simulink model "fuzzy"  (R2024a)
settings: Solver=FixedStepAuto  StartTime=0.0  StopTime=250  FixedStep=1e-2  RelTol=1e-3
InitFcn:
  | % close;
  | % % % z
  | k_p_z = -4;
  | k_i_z = -.5;
  | k_d_z = -8;
  | k_a_z = -2;
  | % %
  | % % % psi
  | k_p_psi = 5.84;
  | k_i_psi = 0;
  | k_d_psi = .836;
  | k_a_psi = 0;
  | % %
  | % % phi
  | k_p_phi = 1;
  | k_d_phi = 0.32;
  | %
  | % % tt
  | k_p_tt = 1;
  | k_d_tt = .302;
  | %
  | % % x
  | k_p_x = -5.99;
  | k_i_x = -2.8;
  | k_d_x = -1.244;
  | k_a_x = -7.94;
  | %
  | % % y
  | k_p_y = 5.99;
  | k_i_y = 2.8;
  | k_d_y = 1.244;
  | k_a_y = 7.94;
StopFcn:
  | plot3(x,y,-z,['b','-'],x_g,y_g,-z_g,['r','--'],'LineWidth',1.25);
  | xlabel('x');
  | ylabel('y');
  | zlabel('z');
  | grid on;
undefined symbols (not defined in the file): k_a_phi, k_a_tt, k_i_phi, k_i_tt
libraries: fuzblock x6, simulink x6
settings Model: Creator=luand  LastModifiedBy=luand
settings DataIOCC: ReturnWorkspaceOutputs=off

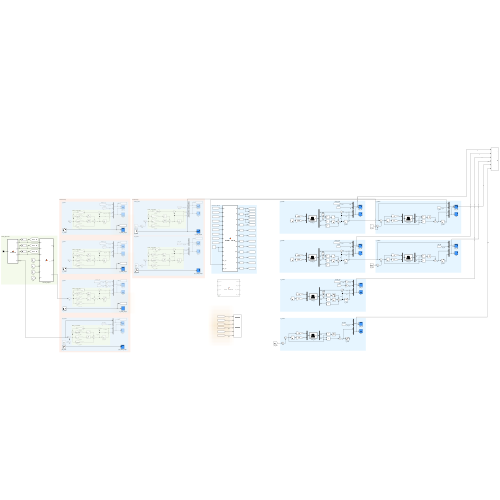
[thumbnail: Simulink's stored preview of the top-level diagram]
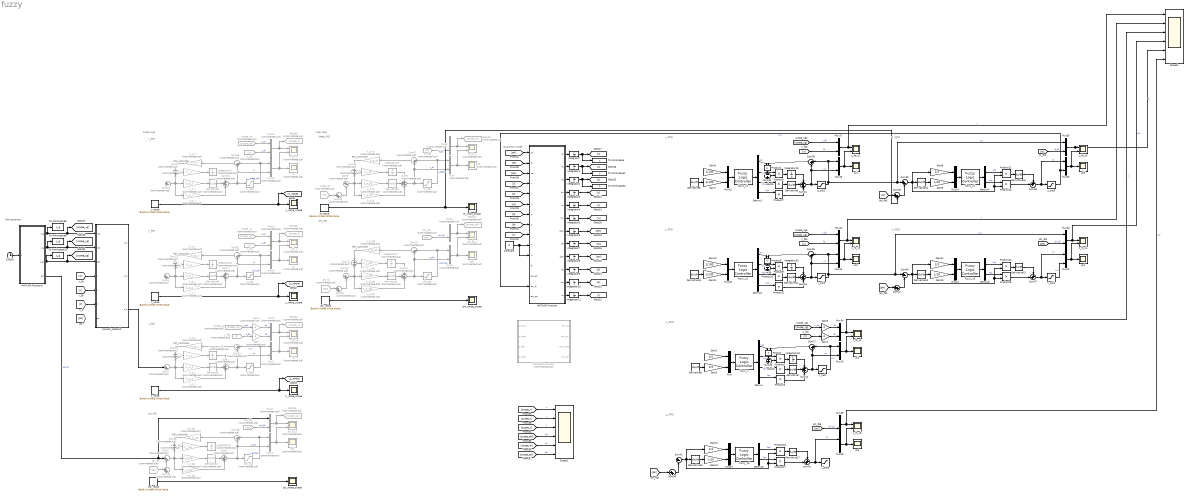
== system fuzzy ==
  note: Path generate
  note: Inner loop
  note: z_PID
  note: PID_controller
  note: PID_controller
  note: psi_PID
  note: Quadrotor Model
  note: PID_controller
  note: PID_controller
  note: PID_controller
  note: PID_controller
  note: theta_PID
  note: phi_PID
  note: Outer loop
  note: y_PID
  note: x_PID
  note: z_FPID
  note: x_FPID
  note: y_FPID
  note: z_FPID
  note: z_FPID
  note: z_FPID
  Clock5 : Clock
  Constant : Constant  Value=0
  Demux : Demux
  Demux1 : Demux
  Demux2 : Demux
  Demux3 : Demux  Outputs=2
  Demux4 : Demux  Outputs=2
  Demux5 : Demux  Outputs=2
  Derivative{,1..5} (6 alike) : Derivative  Commented=on
  Derivative{6..17} (12 alike) : Derivative
  Gain : Gain  Commented=on  Gain=-1
  Gain1 : Gain  Commented=on  Gain=-1
  Gain{6..7,10..11} (4 alike) : Gain  Gain=1/100
  Gain12 : Gain  Gain=1/3
  Gain13 : Gain  Gain=1/10
  Gain14 : Gain  Gain=1/3
  Gain15 : Gain  Gain=1/10
  Gain2 : Gain  Gain=1/5
  Gain3 : Gain  Gain=1/5
  Gain4 : Gain  Gain=-1
  Gain5 : Gain  Gain=-1
  Gain8 : Gain  Gain=1/3
  Gain9 : Gain  Gain=1/10
  Goto24 : Goto  Commented=on  GotoTag=scope_phi
  Goto25 : Goto  Commented=on  GotoTag=scope_y
  Goto26 : Goto  Commented=on  GotoTag=scope_tt
  Goto28 : Goto  Commented=on  GotoTag=scope_psi
  Goto30 : Goto  Commented=on  GotoTag=scope_x
  Goto34 : Goto  Commented=on  GotoTag=scope_z
  Integrator{,1,3..5} (5 alike) : Integrator  LimitOutput=on  UpperSaturationLimit=10000  LowerSaturationLimit=-10000
  Integrator{8..11} (4 alike) : Integrator  LimitOutput=on  UpperSaturationLimit=100  LowerSaturationLimit=-100
  Integrator{12..15,17} (5 alike) : Integrator  Commented=on  LimitOutput=on  UpperSaturationLimit=1000  LowerSaturationLimit=-1000
  Integrator16 : Integrator  Commented=on
  Integrator{6..7,18..20} (5 alike) : Integrator  LimitOutput=on  UpperSaturationLimit=1000  LowerSaturationLimit=-1000
  Integrator2 : Integrator  LimitOutput=on  UpperSaturationLimit=0  LowerSaturationLimit=-1000
  MATLAB Function : MATLAB Function  TreatAsAtomicUnit=on
  MATLAB Function1 : MATLAB Function  Commented=on  TreatAsAtomicUnit=on
  MATLAB Function2 : MATLAB Function  TreatAsAtomicUnit=on
  Mux{,13..29} (18 alike) : Mux  Inputs=2
  Mux{1..12} (12 alike) : Mux  Commented=on  Inputs=2
  Product{,1..17} (18 alike) : Product
  Scope1 : Scope  NumInputPorts=6
  Scope2 : Scope  NumInputPorts=6
  Sum{1,3,7,9,11,33} (6 alike) : Sum  Commented=on  Inputs=+++
  Sum{2,4,6,8,10,12} (6 alike) : Sum  Commented=on  Inputs=|+-
  Sum13 : Sum  Commented=on  Inputs=++|
  Sum14 : Sum  Inputs=+++
  Sum{15,19,22,27,29,32} (6 alike) : Sum  Commented=on  Inputs=|-+
  Sum16 : Sum  Commented=on  Inputs=-|+
  Sum17 : Sum  Inputs=|-+
  Sum18 : Sum  Commented=on  Inputs=+|+
  Sum20 : Sum  Inputs=-|+
  Sum21 : Sum  Commented=on  Inputs=+|+
  Sum23 : Sum  Commented=on  Inputs=|++
  Sum24 : Sum  Inputs=+++
  Sum25 : Sum  Commented=on  Inputs=|++
  Sum26 : Sum  Commented=on  Inputs=+|+
  Sum28 : Sum  Inputs=|-+
  Sum30 : Sum  Inputs=-|+
  Sum31 : Sum  Commented=on  Inputs=-|+
  Sum34 : Sum  Inputs=+++
  Sum35 : Sum  Inputs=|-+
  Sum36 : Sum  Inputs=-|+
  Sum37 : Sum  Inputs=++|
  Sum38 : Sum  Inputs=++|
  Sum39 : Sum  Inputs=|+-
  Sum40 : Sum  Inputs=|+-
  Sum41 : Sum  Inputs=++|
  Sum42 : Sum  Inputs=|+-
  Sum45 : Sum  Inputs=|++
  Sum46 : Sum  Inputs=|++
  Sum47 : Sum  Inputs=|++
  Sum5 : Sum  Commented=on  Inputs=-|+
  To Workspace : ToWorkspace  VariableName=x  SampleTime=-1
      settings: Save2DSignal=2-D array (concatenate along first dimension)
  To Workspace1 : ToWorkspace  VariableName=y  SampleTime=-1
      settings: Save2DSignal=2-D array (concatenate along first dimension)
  To Workspace10 : ToWorkspace  VariableName=z_g  SampleTime=-1
      settings: Save2DSignal=2-D array (concatenate along first dimension)
  To Workspace2 : ToWorkspace  VariableName=z  SampleTime=-1
      settings: Save2DSignal=2-D array (concatenate along first dimension)
  To Workspace8 : ToWorkspace  VariableName=x_g  SampleTime=-1
      settings: Save2DSignal=2-D array (concatenate along first dimension)
  To Workspace9 : ToWorkspace  VariableName=y_g  SampleTime=-1
      settings: Save2DSignal=2-D array (concatenate along first dimension)
  convert_setpoint : MATLAB Function  TreatAsAtomicUnit=on
  fuzzy_z : fuzblock/Fuzzy Logic  Controller  FIS='fuzzy_z.fis'  OutputSampleNumber=11  DataType=double  FuzzifiedInputs=off  RuleFiringStrengths=off  RuleOutputs=off  AggregatedOutputs=off  SimulateUsing=Interpreted execution  OutOfRangeInputValueMessage=warning  NoRuleFiredMessage=warning  EmptyOutputFuzzySetMessage=warning
  fuzzy_z1 : fuzblock/Fuzzy Logic  Controller  FIS='fuzzy_x.fis'  OutputSampleNumber=11  DataType=double  FuzzifiedInputs=off  RuleFiringStrengths=off  RuleOutputs=off  AggregatedOutputs=off  SimulateUsing=Interpreted execution  OutOfRangeInputValueMessage=warning  NoRuleFiredMessage=warning  EmptyOutputFuzzySetMessage=warning
  fuzzy_z2 : fuzblock/Fuzzy Logic  Controller  FIS='fuzzy_y.fis'  OutputSampleNumber=11  DataType=double  FuzzifiedInputs=off  RuleFiringStrengths=off  RuleOutputs=off  AggregatedOutputs=off  SimulateUsing=Interpreted execution  OutOfRangeInputValueMessage=warning  NoRuleFiredMessage=warning  EmptyOutputFuzzySetMessage=warning
  fuzzy_z3 : fuzblock/Fuzzy Logic  Controller  FIS='fuzzy_phi.fis'  OutputSampleNumber=101  DataType=double  FuzzifiedInputs=off  RuleFiringStrengths=off  RuleOutputs=off  AggregatedOutputs=off  SimulateUsing=Interpreted execution  OutOfRangeInputValueMessage=warning  NoRuleFiredMessage=warning  EmptyOutputFuzzySetMessage=warning
  fuzzy_z4 : fuzblock/Fuzzy Logic  Controller  FIS='fuzzy_tt.fis'  OutputSampleNumber=101  DataType=double  FuzzifiedInputs=off  RuleFiringStrengths=off  RuleOutputs=off  AggregatedOutputs=off  SimulateUsing=Interpreted execution  OutOfRangeInputValueMessage=warning  NoRuleFiredMessage=warning  EmptyOutputFuzzySetMessage=warning
  fuzzy_z5 : fuzblock/Fuzzy Logic  Controller  FIS='fuzzy_psi.fis'  OutputSampleNumber=101  DataType=double  FuzzifiedInputs=off  RuleFiringStrengths=off  RuleOutputs=off  AggregatedOutputs=off  SimulateUsing=Interpreted execution  OutOfRangeInputValueMessage=warning  NoRuleFiredMessage=warning  EmptyOutputFuzzySetMessage=warning
  k_a_phi : Gain  Commented=on  Gain=k_a_phi
  k_a_psi : Gain  Commented=on  Gain=k_a_psi
  k_a_tt : Gain  Commented=on  Gain=k_a_tt
  k_a_x : Gain  Commented=on  Gain=k_a_x
  k_a_y : Gain  Commented=on  Gain=k_a_y
  k_a_z : Gain  Commented=on  Gain=k_a_z
  k_d_phi : Gain  Commented=on  Gain=k_d_phi
  k_d_psi : Gain  Commented=on  Gain=k_d_psi
  k_d_tt : Gain  Commented=on  Gain=k_d_tt
  k_d_x : Gain  Commented=on  Gain=k_d_x
  k_d_y : Gain  Commented=on  Gain=k_d_y
  k_d_z : Gain  Commented=on  Gain=k_d_z
  k_i_phi : Gain  Commented=on  Gain=k_i_phi
  k_i_psi : Gain  Commented=on  Gain=k_i_psi
  k_i_tt : Gain  Commented=on  Gain=k_i_tt
  k_i_x : Gain  Commented=on  Gain=k_i_x
  k_i_y : Gain  Commented=on  Gain=k_i_y
  k_i_z : Gain  Commented=on  Gain=k_i_z
  k_p_phi : Gain  Commented=on  Gain=k_p_phi
  k_p_psi : Gain  Commented=on  Gain=k_p_psi
  k_p_tt : Gain  Commented=on  Gain=k_p_tt
  k_p_x : Gain  Commented=on  Gain=k_p_x
  k_p_y : Gain  Commented=on  Gain=k_p_y
  k_p_z : Gain  Commented=on  Gain=k_p_z
  phi_fb : From  Commented=on  GotoTag=phi
  phi_fb1 : From  Commented=on  GotoTag=phi
  phi_fb_u : Scope  Commented=on  NumInputPorts=2
  phi_noise : simulink/Sources/Band-Limited White Noise  Cov=[0.001]  Ts=0.1  seed=[23341]
  phi_noise_scope : Scope
  phi_sat : Saturate  Commented=on  UpperLimit=100  LowerLimit=-100
  psi_fb : From  Commented=on  GotoTag=psi
  psi_fb1 : From  Commented=on  GotoTag=psi
  psi_fb_u : Scope  Commented=on  NumInputPorts=2
  psi_noise : simulink/Sources/Band-Limited White Noise  Cov=[0.0005]  Ts=0.1  seed=[12424]
  psi_noise_scope : Scope
  psi_sat : Saturate  Commented=on  UpperLimit=50  LowerLimit=-50
  scope_xg : From  Commented=on  GotoTag=scope_xg
  scope_yg : From  Commented=on  GotoTag=scope_yg
  scope_zg : From  Commented=on  GotoTag=scope_zg
  theta_fb : From  Commented=on  GotoTag=tt
  tt_fb1 : From  Commented=on  GotoTag=tt
  tt_fb_u : Scope  Commented=on  NumInputPorts=2
  tt_noise : simulink/Sources/Band-Limited White Noise  Cov=[0.001]  Ts=0.1  seed=[23341]
  tt_noise_scope : Scope
  tt_sat : Saturate  Commented=on  UpperLimit=100  LowerLimit=-100
  uphi : Scope  Commented=on
  upsi : Scope  Commented=on
  utt : Scope  Commented=on
  ux : Scope  Commented=on
  uy : Scope  Commented=on
  uz : Scope  Commented=on
  uz{1..6} (6 alike) : Scope
  x_fb1 : From  Commented=on  GotoTag=x
  x_fb_u : Scope  Commented=on  NumInputPorts=2
  x_noise : simulink/Sources/Band-Limited White Noise  Cov=[0.0001]  Ts=0.1  seed=[23341]
  x_noise_scope : Scope
  x_sat : Saturate  Commented=on  UpperLimit=pi/2  LowerLimit=-pi/2
  y_fb1 : From  Commented=on  GotoTag=y
  y_fb_u : Scope  Commented=on  NumInputPorts=2
  y_noise : simulink/Sources/Band-Limited White Noise  Cov=[0.0001]  Ts=0.1  seed=[24432]
  y_noise_scope : Scope
  y_sat : Saturate  Commented=on  UpperLimit=pi/2  LowerLimit=-pi/2
  z_fb1 : From  Commented=on  GotoTag=z
  z_fb_u : Scope  Commented=on  NumInputPorts=2
  z_fb_u{1..6} (6 alike) : Scope  NumInputPorts=2
  z_noise : simulink/Sources/Band-Limited White Noise  Cov=[0.01]  Ts=0.1  seed=[55123]
  z_noise_scope : Scope
  z_sat : Saturate  Commented=on  UpperLimit=40  LowerLimit=0
  z_sat1 : Saturate  UpperLimit=40  LowerLimit=0
  z_sat2 : Saturate  UpperLimit=pi/15  LowerLimit=-pi/15
  z_sat3 : Saturate  UpperLimit=pi/15  LowerLimit=-pi/15
  z_sat4 : Saturate  UpperLimit=100  LowerLimit=-100
  z_sat5 : Saturate  UpperLimit=100  LowerLimit=-100
  z_sat6 : Saturate  UpperLimit=100  LowerLimit=-100
  wires:
  k_a_phi/1 -> Sum21/1
  phi_fb/1 -> Sum23/1
  Sum23/1 -> Sum10/2
  Sum11/1 -> Mux5/2, Sum22/2, phi_sat/1  "u_phi"
  k_d_phi/1 -> Derivative2/1
  phi_fb1/1 -> Mux6/2  "phi_fb"
  Mux5/1 -> uphi/1, phi_fb_u/2
  Mux6/1 -> phi_fb_u/1, Goto24/1
  x_sat/1 -> Mux12/1, Sum29/1  "theta_ref"
  Sum21/1 -> k_i_phi/1
  [r] -> MATLAB Function/9(r)
  MATLAB Function2/4(psi) -> Mux3/1, Sum2/1  "psi_sp"
  phi_noise/1 -> phi_noise_scope/1
  Integrator8/1 -> [psi]
  Sum13/1 -> Sum2/2
  Sum19/1 -> k_a_psi/1
  psi_fb1/1 -> Mux3/2  "psi_fb"
  MATLAB Function/11(dq) -> Integrator10/1
  Mux4/1 -> upsi/1, psi_fb_u/2
  Constant/1 -> MATLAB Function/11(fy), MATLAB Function/10(fx)
  k_a_psi/1 -> Sum18/1
  Mux1/1 -> uz/1, z_fb_u/2
  Mux3/1 -> psi_fb_u/1, Goto28/1
  k_p_psi/1 -> Sum3/3
  Derivative1/1 -> Sum3/2
  Gain/1 -> Mux2/2  "fb"
  Integrator5/1 -> [w]
  [tt] -> MATLAB Function/2(tt)
  Sum22/1 -> k_a_phi/1
  k_p_phi/1 -> Sum11/3
  Integrator/1 -> To Workspace/1, [x]
  psi_sat/1 -> Sum19/1, Mux4/1  "u_psisat"
  MATLAB Function/4(du) -> Integrator3/1
  k_d_psi/1 -> Derivative1/1
  Sum16/1 -> k_i_z/1
  Integrator12/1 -> Sum1/1
  k_a_z/1 -> Sum16/1
  Mux2/1 -> Goto34/1, z_fb_u/1
  Gain1/1 -> Mux2/1  "sp"
  [phi] -> MATLAB Function/1(phi)
  k_d_z/1 -> Derivative/1
  z_noise/1 -> [z_noise], z_noise_scope/1
  Integrator10/1 -> [q]
  k_i_z/1 -> Integrator12/1
  Sum1/1 -> Mux1/2, Sum15/2, z_sat/1  "uz"
  psi_fb/1 -> Sum13/1
  Sum18/1 -> k_i_psi/1
  Derivative2/1 -> Sum11/2
  [psi] -> MATLAB Function/3(psi)
  k_i_phi/1 -> Integrator17/1
  phi_sat/1 -> Mux5/1, Sum22/1  "u_phisat"
  k_i_tt/1 -> Integrator16/1
  k_i_y/1 -> Integrator15/1
  z_sat/1 -> Mux1/1, Sum15/1  "u_z"
  [p] -> MATLAB Function/7(p)
  MATLAB Function/1(dx) -> Integrator/1
  Integrator7/1 -> [tt]
  Sum2/1 -> Sum18/2, k_d_psi/1, k_p_psi/1
  Integrator1/1 -> To Workspace1/1, [y]
  MATLAB Function/2(dy) -> Integrator1/1
  k_i_psi/1 -> Integrator13/1
  Integrator3/1 -> [u]
  Sum3/1 -> psi_sat/1, Sum19/2, Mux4/2  "u_psi"
  Integrator2/1 -> To Workspace2/1, [z]
  [w] -> MATLAB Function/6(w)
  Integrator11/1 -> [r]
  Integrator9/1 -> [p]
  [u] -> MATLAB Function/4(u)
  Integrator6/1 -> [phi]
  MATLAB Function/5(dv) -> Integrator4/1
  psi_noise/1 -> psi_noise_scope/1
  MATLAB Function/6(dw) -> Integrator5/1
  z_fb1/1 -> Gain/1  "z_fb"
  Integrator4/1 -> [v]
  MATLAB Function/12(dr) -> Integrator11/1
  MATLAB Function/9(dpsi) -> Integrator8/1
  [q] -> MATLAB Function/8(q)
  Sum10/1 -> k_d_phi/1, Sum21/2, k_p_phi/1
  [v] -> MATLAB Function/5(v)
  MATLAB Function/10(dp) -> Integrator9/1
  MATLAB Function/8(dtt) -> Integrator7/1
  Sum15/1 -> k_a_z/1
  MATLAB Function/3(dz) -> Integrator2/1
  MATLAB Function/7(dphi) -> Integrator6/1
  Integrator17/1 -> Sum11/1
  theta_fb/1 -> Sum25/1
  Sum25/1 -> Sum8/2
  Integrator16/1 -> Sum9/1
  k_p_tt/1 -> Sum9/3
  Sum26/1 -> k_i_tt/1
  k_d_tt/1 -> Derivative3/1
  Derivative3/1 -> Sum9/2
  k_a_tt/1 -> Sum26/1
  Sum27/1 -> k_a_tt/1
  tt_sat/1 -> Mux7/1, Sum27/1  "u_ttsat"
  y_sat/1 -> Mux9/1, Sum32/1  "phi_ref"
  Mux8/1 -> Goto26/1, tt_fb_u/1
  Mux7/1 -> utt/1, tt_fb_u/2
  tt_fb1/1 -> Mux8/2  "tt_fb"
  Sum9/1 -> Mux7/2, Sum27/2, tt_sat/1  "u_tt"
  tt_noise/1 -> Sum46/2, tt_noise_scope/1
  Sum8/1 -> k_d_tt/1, Sum26/2, k_p_tt/1
  Integrator13/1 -> Sum3/1
  Clock5/1 -> MATLAB Function2/1(t)
  k_d_y/1 -> Derivative4/1
  Integrator15/1 -> Sum7/1
  k_p_y/1 -> Sum7/3
  Sum31/1 -> k_i_y/1
  k_a_y/1 -> Sum31/1
  Sum7/1 -> Mux9/2, Sum32/2, y_sat/1  "uy"
  Sum32/1 -> k_a_y/1
  y_noise/1 -> [y_noise], y_noise_scope/1
  x_noise/1 -> [x_noise], x_noise_scope/1
  Sum29/1 -> k_a_x/1
  Sum33/1 -> x_sat/1, Sum29/2, Mux12/2  "ux"
  k_a_x/1 -> Sum5/1
  Sum5/1 -> k_i_x/1
  k_p_x/1 -> Sum33/3
  Integrator14/1 -> Sum33/1
  k_d_x/1 -> Derivative5/1
  k_i_x/1 -> Integrator14/1
  y_fb1/1 -> Mux10/2  "y_fb"
  Mux10/1 -> Goto25/1, y_fb_u/1
  Mux9/1 -> uy/1, y_fb_u/2
  Mux11/1 -> x_fb_u/1, Goto30/1
  Mux12/1 -> ux/1, x_fb_u/2
  x_fb1/1 -> Mux11/2  "x_fb"
  [scope_x] -> Scope1/1  "x"
  [scope_y] -> Scope1/2  "y"
  [scope_z] -> Scope1/3  "z"
  [scope_psi] -> Scope1/6  "psi"
  [scope_phi] -> Scope1/4  "phi"
  [scope_tt] -> Scope1/5  "tt"
  Derivative4/1 -> Sum7/2
  Derivative5/1 -> Sum33/2
  MATLAB Function2/1(x_g) -> [scope_xg], convert_setpoint/1(xsp), To Workspace8/1
  MATLAB Function2/2(y_g) -> [scope_yg], convert_setpoint/2(ysp), To Workspace9/1
  MATLAB Function2/3(z_g) -> [scope_zg], convert_setpoint/3(zsp), To Workspace10/1
  scope_xg/1 -> Mux11/1  "x_sp"
  scope_zg/1 -> Gain1/1  "z_sp"
  scope_yg/1 -> Mux10/1  "y_sp"
  [x] -> convert_setpoint/4(x)
  [y] -> convert_setpoint/5(y)
  [z] -> convert_setpoint/6(z)
  Sum4/1 -> Sum16/2, k_p_z/1, k_d_z/1
  Sum12/1 -> Sum5/2, k_p_x/1, k_d_x/1
  Sum6/1 -> Sum31/2, k_p_y/1, k_d_y/1
  Derivative/1 -> Sum1/2
  Derivative6/1 -> Gain3/1
  Gain2/1 -> Mux/1
  Gain3/1 -> Mux/2
  Derivative7/1 -> Sum14/2
  z_sat1/1 -> Mux13/1, Sum17/1  "u_z"
  Sum14/1 -> z_sat1/1, Mux13/2, Sum17/2  "uz"
  Product1/1 -> Integrator18/1
  Product2/1 -> Derivative7/1
  Integrator18/1 -> Sum14/1
  fuzzy_z/1 -> Demux/1
  Product/1 -> Sum20/1
  Demux/3 -> Product2/1  "kdz"
  Demux/4 -> Product3/1  "kpz"
  Product3/1 -> Sum14/3
  Mux/1 -> fuzzy_z/1
  k_p_z/1 -> Sum1/3
  Demux/2 -> Product1/1  "kiz"
  Sum20/1 -> Product1/2
  Demux/1 -> Product/1  "kaz"
  Sum17/1 -> Product/2
  convert_setpoint/3(z_b) -> Sum4/1
  [scope_zg] -> Gain5/1  "x_fb"
  [z] -> Gain4/1
  Gain5/1 -> Mux14/1  "sp"
  Mux14/1 -> Scope2/3, z_fb_u1/1  "z"
  Gain4/1 -> Mux14/2  "fb"
  Mux13/1 -> uz1/1, z_fb_u1/2
  Mux16/1 -> z_fb_u2/2, uz2/1
  [x] -> Mux17/2  "fb"
  Mux17/1 -> Scope2/1, z_fb_u2/1  "x"
  [scope_xg] -> Mux17/1  "x_fb"
  Sum28/1 -> Product4/2
  Demux1/1 -> Product4/1  "kaz"
  Sum30/1 -> Product5/2
  Demux1/2 -> Product5/1  "kiz"
  Mux15/1 -> fuzzy_z1/1
  Product7/1 -> Sum24/3
  Demux1/4 -> Product7/1  "kpz"
  Demux1/3 -> Product6/1  "kdz"
  Product4/1 -> Sum30/1
  fuzzy_z1/1 -> Demux1/1
  Integrator19/1 -> Sum24/1
  Product6/1 -> Derivative9/1
  Product5/1 -> Integrator19/1
  Sum24/1 -> Sum28/2, Mux16/2, z_sat2/1  "uz"
  z_sat2/1 -> Mux26/1, Sum39/1, Mux16/1, Sum28/1  "u_z"
  Derivative9/1 -> Sum24/2
  Gain7/1 -> Mux15/2
  Gain6/1 -> Mux15/1
  Derivative8/1 -> Gain7/1
  Derivative10/1 -> Gain11/1
  Gain10/1 -> Mux18/1
  Gain11/1 -> Mux18/2
  Derivative11/1 -> Sum34/2
  z_sat3/1 -> Mux23/1, Sum40/1, Sum35/1, Mux19/1  "u_z"
  Sum34/1 -> z_sat3/1, Mux19/2, Sum35/2  "uz"
  Product9/1 -> Integrator20/1
  Product10/1 -> Derivative11/1
  Integrator20/1 -> Sum34/1
  fuzzy_z2/1 -> Demux2/1
  Product8/1 -> Sum36/1
  Demux2/3 -> Product10/1  "kdz"
  Demux2/4 -> Product11/1  "kpz"
  Product11/1 -> Sum34/3
  Mux18/1 -> fuzzy_z2/1
  Demux2/2 -> Product9/1  "kiz"
  Sum36/1 -> Product9/2
  Demux2/1 -> Product8/1  "kaz"
  Sum35/1 -> Product8/2
  [scope_yg] -> Mux20/1  "x_fb"
  Mux20/1 -> Scope2/2, z_fb_u3/1  "y"
  [y] -> Mux20/2  "fb"
  Mux19/1 -> uz3/1, z_fb_u3/2
  Mux22/1 -> z_fb_u4/2, uz4/1
  Sum40/1 -> Gain14/1, Derivative12/1, Product14/2, Product15/2
  Mux21/1 -> fuzzy_z3/1
  Demux3/2 -> Product15/1  "kpz"
  Demux3/1 -> Product14/1  "kdz"
  fuzzy_z3/1 -> Demux3/1
  Product14/1 -> Derivative13/1
  Sum37/1 -> Mux22/1, z_sat4/1  "uz"
  z_sat4/1 -> Mux22/2  "u_z"
  Gain15/1 -> Mux21/2
  Gain14/1 -> Mux21/1
  Derivative12/1 -> Gain15/1
  Mux26/1 -> Scope2/5, z_fb_u5/1  "tt"
  Mux23/1 -> Scope2/4, z_fb_u4/1  "phi"
  Derivative13/1 -> Sum37/1
  Product15/1 -> Sum37/2
  Product13/1 -> Sum38/2
  Derivative15/1 -> Sum38/1
  Derivative14/1 -> Gain9/1
  Gain8/1 -> Mux24/1
  Gain9/1 -> Mux24/2
  Sum38/1 -> z_sat5/1, Mux25/1  "uz"
  Product12/1 -> Derivative15/1
  fuzzy_z4/1 -> Demux4/1
  Demux4/1 -> Product12/1  "kdz"
  Demux4/2 -> Product13/1  "kpz"
  Mux24/1 -> fuzzy_z4/1
  Sum39/1 -> Product13/2, Product12/2, Derivative14/1, Gain8/1
  Mux25/1 -> uz5/1, z_fb_u5/2
  z_sat5/1 -> Mux25/2, MATLAB Function/14(tau_tt)  "u_z"
  [tt] -> Mux26/2  "tt_fb"
  [phi] -> Mux23/2  "phi_fb"
  [psi] -> Mux29/2  "phi_fb"
  Product17/1 -> Sum41/2
  Derivative17/1 -> Sum41/1
  Derivative16/1 -> Gain13/1
  Gain12/1 -> Mux27/1
  Gain13/1 -> Mux27/2
  Sum41/1 -> z_sat6/1, Mux28/1  "uz"
  Product16/1 -> Derivative17/1
  fuzzy_z5/1 -> Demux5/1
  Demux5/1 -> Product16/1  "kdz"
  Demux5/2 -> Product17/1  "kpz"
  Mux27/1 -> fuzzy_z5/1
  Sum42/1 -> Product17/2, Product16/2, Derivative16/1, Gain12/1
  Mux28/1 -> uz6/1, z_fb_u6/2
  Mux29/1 -> Scope2/6, z_fb_u6/1  "psi"
  [psi] -> Sum45/1
  Sum45/1 -> Sum42/2
  [tt] -> Sum46/1
  Sum46/1 -> Sum39/2
  [phi] -> Sum47/1
  Sum47/1 -> Sum40/2

== matlab function fuzzy/MATLAB Function1 ==
  data: fthrust output; tau_phi output; tau_theta output; tau_psi output; p_front input; p_back input; p_left input; p_right input
function [fthrust, tau_phi, tau_theta, tau_psi] = Motor_dynamics(p_front, p_back, p_left, p_right)

fthrust = k_thrust*(p_front+p_back+p_left+p_right);
tau_phi = l*k_thrust*(-p_right+p_left);
tau_theta = l*k_thrust*(p_front+p_back);
tau_psi = k_momen*(-p_front-p_back+p_left+p_right);

== matlab function fuzzy/MATLAB Function ==
  data: phi input; tt input; psi input; u input; dx output; v input; w input; p input; q input; r input; fx input; fy input; fz input; tau_phi input; tau_tt input; tau_psi input; dy output; dz output; du output; dv output; dw output; dphi output; dtt output; dpsi output; dp output; dq output; dr output
function [dx,dy,dz,du,dv,dw,dphi,dtt,dpsi,dp,dq,dr]=Dynamics_plustype(phi,tt,psi,u,v,w,p,q,r,fx,fy,fz,tau_phi,tau_tt,tau_psi)

% Eqs. 16-19

M = 1.2;
m = .075;
g = 9.81;
R = .1;
l = .22;

Jx = .4*M*R*R+2*l*l*m;
Jy = .4*M*R*R+2*l*l*m;
Jz = .4*M*R*R+4*l*l*m;

dx = cos(tt)*cos(psi)*u+(sin(phi)*sin(tt)*cos(psi)-cos(phi)*sin(psi))*v+(cos(phi)*sin(tt)*cos(psi)+sin(phi)*sin(psi))*w;
dy = cos(tt)*sin(psi)*u+(sin(phi)*sin(tt)*sin(psi)+cos(phi)*cos(psi))*v+(cos(phi)*sin(tt)*sin(psi)-sin(phi)*cos(psi))*w;
dz = -(sin(tt)*u-sin(phi)*cos(tt)*v-cos(phi)*cos(tt)*w);

du = (r*v-q*w)-g*sin(tt);
dv = (p*w-r*u)+g*cos(tt)*sin(phi);
dw = (q*u-p*v)+g*cos(tt)*cos(phi)-fz/(M+4*m);

dphi = p+sin(phi)*tan(phi)*q+cos(phi)*tan(tt)*r;
dtt  = cos(phi)*q-sin(phi)*r;
dpsi = sin(phi)*q/cos(tt)+cos(phi)*r/cos(tt);

dp = ((Jy-Jz)*q*r+tau_phi)/Jx;
dq = ((Jz-Jx)*p*r+tau_tt)/Jy;
dr = ((Jx-Jy)*q*p+tau_psi)/Jz;

== matlab function fuzzy/MATLAB Function2 ==
  data: t input; x_g output; y_g output; z_g output; psi output
function [x_g,y_g,z_g,psi] = path_ground(t)

% psi = 100-100*exp(-.02*t);
psi = 0;
% psi = sin(.3*t);
% psi = t/2;

% x_g=0;
% y_g=0;
% if t<30
%     z_g = -10;
% elseif t<70
%     z_g = -20;
% elseif t<100
%     z_g = -30;
% else
%     z_g = 0;
% end

% A = 10; % x range
% a = 5; % grid x
% B = 10; % y range
% b = 4; % grid y
% C = 10;% z range 
% coef = .07;
% x_g = (A-.2*exp(-.014*(t-279.4)))*cos(a*coef*t);
% y_g = (B-.2*exp(-.014*(t-279.4)))*sin(b*coef*t);
% z_g = -C*(1-exp(-5*coef*t));%-sin(.3*t)*sin(.3*t);

% z_g = -C*(1-exp(-.03*t));

% A = 20; % x range
% a = 5; % grid x
% B = 20; % y range
% b = 4; % grid y
% C = 10;% z range 
% coef = .07;
% x_g = (10-.2*exp(-.014*(t-279.4)))*cos(a*coef*t);
% y_g = (10-.2*exp(-.014*(t-279.4)))*sin(b*coef*t);
% % z_g = -10; % dont know why step Z work
% % z_g = -(10-.2*exp(-.014*(t-279.4)));
% z_g = -(10-10*exp(-.05*t));

if t<25
    x_g = 1*t/25;
    y_g = 1*t/25;
    z_g = -3-2*t/25;
elseif t<50
    x_g = 1+(t-25)/25;
    y_g = 1;
    z_g = -5-2*(t-25)/25;
elseif t<75
    x_g = 2;
    y_g = 1+(t-50)/25;
    z_g = -7-2*(t-50)/25;
elseif t<100
    x_g = 2-3*(t-75)/25;
    y_g = 2+(t-75)/25;
    z_g = -9-2*(t-75)/25;
elseif t<125
    x_g = -1;
    y_g = 3-4*(t-100)/25;
    z_g = -11-2*(t-100)/25;
elseif t<150
    x_g = -1+4*(t-125)/25;
    y_g = -1;
    z_g = -13-2*(t-125)/25;
elseif t<175
    x_g = 3-2*(t-150)/25;
    y_g = -1+5*(t-150)/25;
    z_g = -15-2*(t-150)/25;
else
    x_g = 1-min(1,1*(t-175)/25);
    y_g = 4-min(4,4*(t-175)/25);
    z_g = -17+min(16,16*(t-175)/25);
end

% if t<50
%     a=2*exp(.05*(t-50));
%     b=2;
% elseif t<100
%     a=2+exp(.05*(t-100));
%     b=3;
% elseif t<150
%     a=3+exp(.05*(t-150));
%     b=4;
% else
%     b=4*(exp(.02*(150-t)));
%     a=4+4*exp(.1*(t-200));
% end
% z_g = -2*b;
% x_g = a*cos(.5*t);
% y_g = a*sin(.5*t);

== matlab function fuzzy/convert_setpoint ==
  data: xsp input; x_b output; y_b output; ysp input; zsp input; x input; y input; z input; psi input; z_b output
% Ground setpoint to body
function [x_b,y_b,z_b] = convert_setpoint(xsp,ysp,zsp,x,y,z,psi)
xyz_sp_g = [xsp ysp zsp 1];

% R_body_to_ground = [cos(psi)*cos(theta) cos(psi)*sin(theta)*sin(phi)-sin(psi)*cos(phi) cos(psi)*sin(theta)*cos(phi)+sin(psi)*sin(phi);
%                     sin(psi)*cos(theta) sin(psi)*sin(theta)*sin(phi)+cos(psi)*cos(phi) sin(psi)*sin(theta)*cos(phi)-cos(psi)*sin(phi);
%                     -sin(theta) cos(theta)*sin(phi) cos(theta)*cos(phi)];
% P_body_to_ground = [x y z]';
% % T_body_to_ground = [R_body_to_ground P_body_to_ground; 0 0 0 1];
% 
% P_ground_to_body = [-P_body_to_ground'*R_body_to_ground(:,1);
%                     -P_body_to_ground'*R_body_to_ground(:,2);
%                     -P_body_to_ground'*R_body_to_ground(:,3)];
% T_ground_to_body = [R_body_to_ground' P_ground_to_body; 0 0 0 1];
% 
% xyz_sp_b = T_ground_to_body*xyz_sp_g';
% 
% x_b = xyz_sp_b(1);
% y_b = xyz_sp_b(2);
% z_b = xyz_sp_b(3);

R_body_to_ground = [cos(psi) -sin(psi) 0;
                    sin(psi) cos(psi) 0;
                    0 0 1];
P_body_to_ground = [x y z];
P_ground_to_body = [-P_body_to_ground*R_body_to_ground(:,1);
                    -P_body_to_ground*R_body_to_ground(:,2);
                    -P_body_to_ground*R_body_to_ground(:,3)];
T_ground_to_body = [R_body_to_ground' P_ground_to_body; 0 0 0 1];
xyz_sp_b = T_ground_to_body*xyz_sp_g';

x_b = xyz_sp_b(1);
y_b = xyz_sp_b(2);
z_b = xyz_sp_b(3);
